simulink model "cosine_trigger_6_pulse_Closed_loop_1_"  (R2025a)
settings: Solver=VariableStepAuto  StartTime=0.0  StopTime=10  RelTol=1e-3
libraries: spsACVoltageSourceLib x3, spsDCMachineLib x1, spsDCVoltageSourceLib x1, spsGroundLib x1, spsUniversalBridgeLib x1, sps_lib x1
settings Model: Creator=arpit  LastModifiedBy=aditl

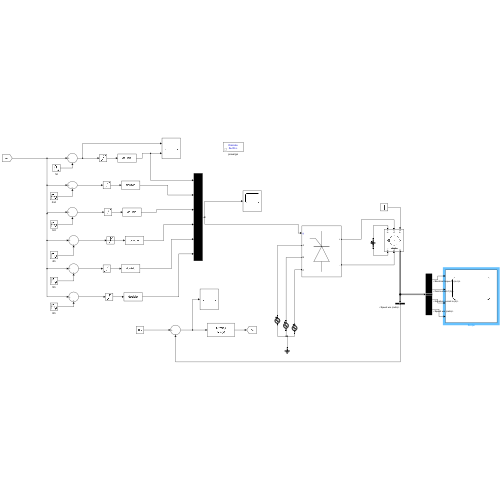
[thumbnail: Simulink's stored preview of the top-level diagram]
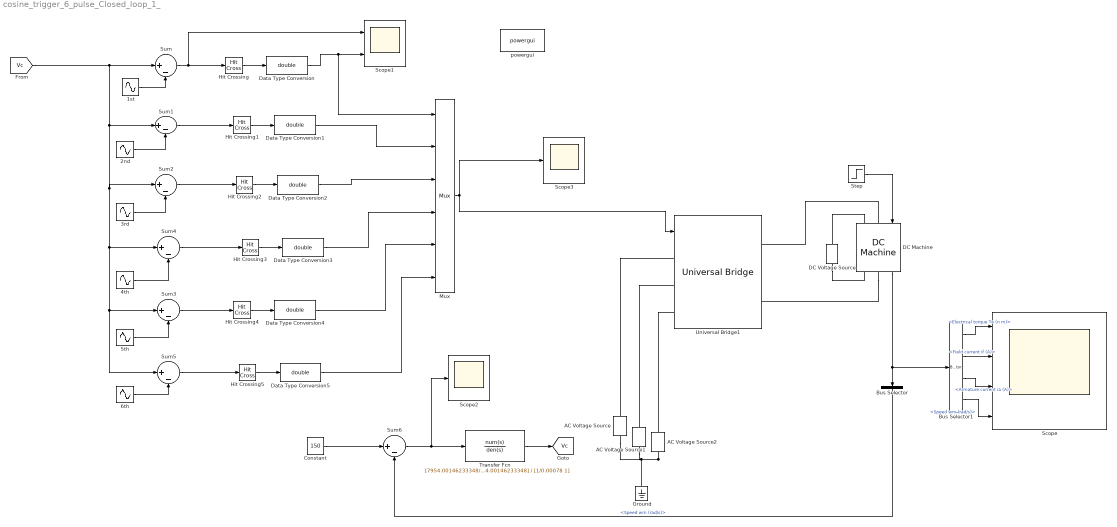
== system cosine_trigger_6_pulse_Closed_loop_1_ ==
  1st : Sin  Amplitude=240  Frequency=2*pi*50  Phase=pi/3  SampleTime=5e-05
  2nd : Sin  Amplitude=240  Frequency=2*pi*50  SampleTime=5e-05
  3rd : Sin  Amplitude=240  Frequency=2*pi*50  Phase=-pi/3  SampleTime=5e-05
  4th : Sin  Amplitude=240  Frequency=2*pi*50  Phase=-2*pi/3  SampleTime=5e-05
  5th : Sin  Amplitude=240  Frequency=2*pi*50  Phase=pi  SampleTime=5e-05
  6th : Sin  Amplitude=240  Frequency=2*pi*50  Phase=2*pi/3  SampleTime=5e-05
  AC Voltage Source : spsACVoltageSourceLib/AC Voltage Source  Amplitude=240  Phase=0  Frequency=50  SampleTime=5e-05  Measurements=None  BusType=swing  Pref=10e3  Qref=0  Qmin=-inf  Qmax=+inf
  AC Voltage Source1 : spsACVoltageSourceLib/AC Voltage Source  Amplitude=240  Phase=-120  Frequency=50  SampleTime=5e-05  Measurements=None  BusType=swing  Pref=10e3  Qref=0  Qmin=-inf  Qmax=+inf
  AC Voltage Source2 : spsACVoltageSourceLib/AC Voltage Source  Amplitude=240  Phase=120  Frequency=50  SampleTime=5e-05  Measurements=None  BusType=swing  Pref=10e3  Qref=0  Qmin=-inf  Qmax=+inf
  Bus Selector : BusSelector  OutputSignals=Speed wm (rad/s)
  Bus Selector1 : BusSelector  OutputSignals=Electrical torque Te (n m),Field current if (A),Armature current ia (A),Speed wm (rad/s)
  Constant : Constant  Value=150
  DC Machine : spsDCMachineLib/DC Machine  PresetModel=02: 5HP 240V 1750RPM Field:150V  MechanicalLoad=Torque TL  FieldType=Wound  ShowDetailedParameters=on  MeasurementBus=off  RLa=[0.78 0.016]  RLf=[150 112.5]  Laf=1.234  MachineConstant=Torque constant (N.m/A)  Ke=1.8  Kt=1.8  J=0.05  Bm=0.01  Tf=0  w0=0  Ifinit=1  TsPowergui=0  TsBlock=-1
  DC Voltage Source : spsDCVoltageSourceLib/DC Voltage Source  Amplitude=150  Measurements=None
  Data Type Conversion{,1..5} (6 alike) : DataTypeConversion  OutDataTypeStr=double  SaturateOnIntegerOverflow=off  RndMeth=Floor
  Ground : spsGroundLib/Ground  LConnTagsString=a
  Hit Crossing{,1..5} (6 alike) : HitCross  HitCrossingDirection=rising
  Mux : Mux  Inputs=6
  Scope : Scope  NumInputPorts=4
      settings: ActiveDisplayYMinimum=-33.118843361629011  ActiveDisplayYMaximum=298.03521918086295
  Scope1 : Scope  NumInputPorts=2
      settings: ActiveDisplayYMinimum=-10317.505107577075  ActiveDisplayYMaximum=93176.067968128744
  Scope2 : Scope
      settings: ActiveDisplayYMinimum=-45.23464  ActiveDisplayYMaximum=116.60497
  Scope3 : Scope
      settings: ActiveDisplayYMinimum=-0.12499999999999997  ActiveDisplayYMaximum=1.125
  Step : Step  Time=5  After=50  SampleTime=0
  Sum{,1..6} (7 alike) : Sum  Inputs=|+-
  Transfer Fcn : TransferFcn  Numerator=[7954.00146233348/4 7954.00146233348]  Denominator=[1/0.00078 1]
  Universal Bridge1 : spsUniversalBridgeLib/Universal Bridge  Arms=3  SnubberResistance=1e5  SnubberCapacitance=inf  Device=Thyristors  Ron=1e-3  Lon=0  ForwardVoltages="[  0  0  ]"  ForwardVoltage=0  GTOparameters=[ 10e-6 , 20e-6 ]  IGBTparameters=[ 1e-6 , 2e-6 ]  Measurements=None  Measurements_2=None  converterType=Rectifier
  powergui : sps_lib/powergui  Priority=1  SimulationMode=Discrete  SampleTime=5e-05  frequency=60  Iterations=50  frequencyindice=50  Pbase=100e6  ErrMax=1e-4  UnitsV=kV  UnitsW=MW  buscounter=0  FunctionMessages=off  echomessages=off  EnableUseOfTLC=off  CurrentSourceSwitches=off  DisableSnubberDevices=off  DisableRonSwitches=off  DisableVfSwitches=off  DisplayEquations=off  AutomaticDiscreteSolvers=off  SolverType=Tustin/Backward Euler (TBE)  Interpol=off  ExternalGateDelay=off  methode=off  Ts=100  x0status=blocks  SPID=on  SwTol=0  HookPort=off  NonlinearTolerance=1e-4  nMaxIteration=100  ContinueOnMaxIteration=off  RestoreLinks=warning  ResistiveCurrentMeasurement=off  Frange=[0:2:500]  Ylog=off  Xlog=on  ShowGrid=off  save=off  variable=ZData  structure=0  ZoomFFT=off  StartTime=0.0  cycles=1  DisplayStyle=1  fundamental=60  FreqAxis=off  MaxFrequency=1000  frequencyindicesteady=1  RmsSteady=1  display=off
  tag scope: Vc=global
  wires:
  Data Type Conversion3/1 -> Mux/4
  Sum2/1 -> Hit Crossing2/1
  Hit Crossing/1 -> Data Type Conversion/1
  Hit Crossing3/1 -> Data Type Conversion3/1
  Data Type Conversion2/1 -> Mux/3
  Data Type Conversion/1 -> Mux/1, Scope1/2
  Hit Crossing1/1 -> Data Type Conversion1/1
  Data Type Conversion5/1 -> Mux/6
  Sum1/1 -> Hit Crossing1/1
  Sum5/1 -> Hit Crossing5/1
  Data Type Conversion4/1 -> Mux/5
  [Vc] -> Sum1/1, Sum2/1, Sum3/1, Sum5/1, Sum4/1, Sum/1
  Sum/1 -> Hit Crossing/1, Scope1/1
  Data Type Conversion1/1 -> Mux/2
  Hit Crossing5/1 -> Data Type Conversion5/1
  3rd/1 -> Sum2/2
  1st/1 -> Sum/2
  5th/1 -> Sum3/2
  4th/1 -> Sum4/2
  2nd/1 -> Sum1/2
  Mux/1 -> Universal Bridge1/1, Scope3/1
  Sum3/1 -> Hit Crossing4/1
  Sum4/1 -> Hit Crossing3/1
  Hit Crossing2/1 -> Data Type Conversion2/1
  6th/1 -> Sum5/2
  Hit Crossing4/1 -> Data Type Conversion4/1
  DC Machine/1 -> Bus Selector/1, Bus Selector1/1
  Sum6/1 -> Scope2/1, Transfer Fcn/1
  Transfer Fcn/1 -> [Vc]
  Bus Selector/1 -> Sum6/2  "<Speed wm (rad/s)>"
  Bus Selector1/1 -> Scope/1  "<Electrical torque Te (n m)>"
  Bus Selector1/2 -> Scope/2  "<Field current if (A)>"
  Bus Selector1/3 -> Scope/3  "<Armature current ia (A)>"
  Bus Selector1/4 -> Scope/4  "<Speed wm (rad/s)>"
  Step/1 -> DC Machine/1
  Constant/1 -> Sum6/1
  connections:
  AC Voltage Source2/LConn1 -- Ground/LConn1 -- AC Voltage Source/LConn1 -- AC Voltage Source1/LConn1
  AC Voltage Source1/RConn1 -- Universal Bridge1/LConn2
  AC Voltage Source/RConn1 -- Universal Bridge1/LConn1
  AC Voltage Source2/RConn1 -- Universal Bridge1/LConn3
  DC Machine/LConn1 -- Universal Bridge1/RConn1
  DC Machine/RConn1 -- Universal Bridge1/RConn2
  DC Voltage Source/LConn1 -- DC Machine/RConn2
  DC Voltage Source/RConn1 -- DC Machine/LConn2
